simulink model "RobotAndBall"  (R2019b)
settings: Solver=VariableStepAuto  StartTime=0.0  StopTime=30  MaxStep=updateFrequency  RelTol=1e-3
values from neighbouring files (symbols this model uses):
  g = bTraj.GoalOnRight    [Launch_Game_TwoRobots.m]
  pOpponentSidePoint = [2.4;0;0.02]'    [Launch_Game_TwoRobots.m]
  Robot1 = RobotPlayer2(initialQ,TransMat1,DistToTable,'Left')    [Launch_Game_TwoRobots.m]
undefined symbols (not defined in the file or in its folder): Ball, Contact_Forces, currentTime, Environment, Net, Robots, Table, tHit, wayPoints, X, Y, Z
libraries: sm_lib x217, nesl_utility x89, Contact_Forces_Lib x8, robotmaniplib x8, Parts_Lib x6, Multibody_Parts_Lib x2, OpenManipulatorLib x1
(part 1 of 7)
settings Model: EnablePacing=on  Creator=Fadi  LastModifiedBy=Fadi
settings DebuggingCC: UnderSpecifiedDimensionMsg=warning
settings DiagnosticsConfigSet: SimMechanicsRigidlyBoundBlock=warning
settings ExplorerConfigSet: InternalSimMechanicsExplorerSettings="<ExplorerConfiguration><canonicalview>default</canonicalview><AnimationSetting><BasePlaybackSpeed>1.0</BasePlaybackSpeed><PlaybackSpeedFactor>1.0</PlaybackSpeedFactor></AnimationSetting><TilePanel><TileInfo><Tiles Columns=\"1\" Count=\"1\" Rows=\"1\"><Column Weight=\"1\"/><Row Weight=\"1\"/><Tile Height=\"1\" Width=\"1\" X=\"0\" Y=\"0\"/></Tiles></TileInfo><SceneInfo><SceneViewer><BGColor><R>0.800000011920928955</R><G>0.800000011920928955</G><B>0.800000011920928955</B></BGColor><Camera><DoPerspective>off</DoPerspective><Position><X>2.72315971629590692</X><Y>-1.50834696696562665</Y><Z>1.58535918834610445</Z></Position><Center><X>1.47795530502201444</X><Y>0.925758447867804257</Y><Z>-0.104613396829873029</Z></Center><Up><X>-0.0499239114255342065</X><Y>0.5522402253466272</Y><Z>0.832188882752636694</Z></Up><ViewLimDist>1</ViewLimDist><YLim>1.3965979297788147</YLim><XLim>2.09410606911342079</XLim></Camera></SceneViewer></SceneInfo></TilePanel><MechEditorPanel><Cameras><Camera><Id>Camera1</Id><Value><Name>Camera1</Name><NativeCamera><PositionTrackingFeature>Subsystem2.wall.R</PositionTrackingFeature><CenterTrackingFeature>Subsystem2.Sphere1.R</CenterTrackingFeature><UpVectorTrackingFeature>Subsystem2.Trans_Table_1.B</UpVectorTrackingFeature><CenterTrackingOrigin>on</CenterTrackingOrigin><UpVectorTrackingDirection>+Z</UpVectorTrackingDirection></NativeCamera></Value></Camera><Camera><Id>Camera2</Id><Value><Name>Camera2</Name><NativeCamera><PositionTrackingFeature>Subsystem2.Trans_Camera.F</PositionTrackingFeature><CenterTrackingFeature>Subsystem2.Sphere1.Sphere.R</CenterTrackingFeature><UpVectorTrackingFeature>Subsystem2.Subsystem1_Bottom</UpVectorTrackingFeature><CenterTrackingOrigin>on</CenterTrackingOrigin><UpVectorTrackingDirection>+Z</UpVectorTrackingDirection></NativeCamera></Value></Camera><Camera><Id>Camera3</Id><Value><Name>Camera3</Name><NativeCamera><PositionKeyframeSet><Keyframe><Time>0.092181068332948451</Time><Value><X>0.74195184319358032</X><Y>-2.1572930074306607</Y><Z>0.99365309767099308</Z></Value></Keyframe><Keyframe><Time>0.51650682316294461</Time><Value><X>1.9459936990787221</X><Y>-2.2708727878259349</Y><Z>1.6833699233296544</Z></Value></Keyframe><Keyframe><Time>0.91598798928248681</Time><Value><X>2.4643039101880788</X><Y>-0.44601289764194951</Y><Z>1.9211952797348746</Z></Value></Keyframe><Keyframe><Time>1.2186543181176928</Time><Value><X>3.2021539618459673</X><Y>0.10402512519052465</Y><Z>4.0341557316442129</Z></Value></Keyframe><Keyframe><Time>1.6120180307329675</Time><Value><X>1.47658917689103</X><Y>0.12690724272667403</Y><Z>3.9442623812733499</Z></Value></Keyframe></PositionKeyframeSet><CenterKeyframeSet><Keyframe><Time>0.092181068332948451</Time><Value><X>1.6664706896861596</X><Y>0.49901858600439208</Y><Z>0.12540780922655559</Z></Value></Keyframe><Keyframe><Time>0.51650682316294461</Time><Value><X>1.8354146075452522</X><Y>-0.67058112685808369</Y><Z>0.88017967418294973</Z></Value></Keyframe><Keyframe><Time>0.91598798928248681</Time><Value><X>1.6687021386666459</X><Y>0.49771837800342772</Y><Z>1.0348366085782759</Z></Value></Keyframe><Keyframe><Time>1.2186543181176928</Time><Value><X>1.8941663009838337</X><Y>1.0681539209099937</Y><Z>2.2215197753492841</Z></Value></Keyframe><Keyframe><Time>1.6120180307329675</Time><Value><X>1.47658917689103</X><Y>0.12690724272667403</Y><Z>-6.705520583238922e-10</Z></Value></Keyframe></CenterKeyframeSet><UpVectorKeyframeSet><Keyframe><Time>0.092181068332948451</Time><Value><X>-0.1061284820573538</X><Y>0.34211066924335759</Y><Z>0.93364716852034846</Z></Value></Keyframe><Keyframe><Time>0.51650682316294461</Time><Value><X>-0.21697539420554568</X><Y>0.42586969042681183</Y><Z>0.87838299453320468</Z></Value></Keyframe><Keyframe><Time>0.91598798928248681</Time><Value><X>-0.56097267127192785</X><Y>0.26399229177590544</Y><Z>0.78461310973558329</Z></Value></Keyframe><Keyframe><Time>1.2186543181176928</Time><Value><X>-0.77959242063363499</X><Y>0.10360787466061416</Y><Z>0.61765772560448062</Z></Value></Keyframe><Keyframe><Time>1.6120180307329675</Time><Value><X>-0.99999555996270595</X><Y>0.0029799420924429784</Y><Z>0</Z></Value></Keyframe></UpVectorKeyframeSet></NativeCamera></Value></Camera><Camera><Id>Camera4</Id><Value><Name>Camera4</Name><NativeCamera><PositionKeyframeSet><Keyframe><Time>0</Time><Value><X>1.634718226767613</X><Y>-3.0526201016665979</Y><Z>0.41798822769624983</Z></Value></Keyframe><Keyframe><Time>0.89165574668215009</Time><Value><X>1.7924264462253023</X><Y>-0.98308392755206742</Y><Z>0.55318583463515325</Z></Value></Keyframe><Keyframe><Time>1.6293434090182939</Time><Value><X>2.0909308885157523</X><Y>1.4458285342327477</Y><Z>2.7042868818040096</Z></Value></Keyframe><Keyframe><Time>2.0068297485509734</Time><Value><X>1.1851088199232986</X><Y>1.7025785749793547</Y><Z>1.9663502501044083</Z></Value></Keyframe><Keyframe><Time>2.3788243854617517</Time><Value><X>-0.73689322282398173</X><Y>1.0135139680640644</Y><Z>0.55257028629247507</Z></Value></Keyframe><Keyframe><Time>2.571358268924163</Time><Value><X>-0.88936881541680146</X><Y>0.54692833301781496</Y><Z>0.20169970252396985</Z></Value></Keyframe><Keyframe><Time>3.0017917048799663</Time><Value><X>-0.99378101342593106</X><Y>-0.88477660537923308</Y><Z>0.55083326620273587</Z></Value></Keyframe><Keyframe><Time>3.8286861711482381</Time><Value><X>1.7669783801752301</X><Y>-0.30065490623969737</Y><Z>0.48883711225906146</Z></Value></Keyframe><Keyframe><Time>4.2649999999999997</Time><Value><X>1.2845531289756482</X><Y>-1.1935311565853732</Y><Z>0.063513925983704644</Z></Value></Keyframe><Keyframe><Time>4.6495452085974227</Time><Value><X>1.2791670874978069</X><Y>-2.7978972452371327</Y><Z>0.18868794730739935</Z></Value></Keyframe><Keyframe><Time>4.9000000000000004</Time><Value><X>1.2995425546894361</X><Y>-3.357189246478486</Y><Z>0.070455084598260581</Z></Value></Keyframe><Keyframe><Time>5.6950000000000003</Time><Value><X>1.766827835394553</X><Y>-3.3830579189989827</Y><Z>0.16082327479556113</Z></Value></Keyframe></PositionKeyframeSet><CenterKeyframeSet><Keyframe><Time>0</Time><Value><X>1.6509000609385884</X><Y>-1.1240589910676677</Y><Z>0.40348620051772122</Z></Value></Keyframe><Keyframe><Time>0.89165574668215009</Time><Value><X>0.93615742103789701</X><Y>-0.20137995272314729</Y><Z>0.37829480091806594</Z></Value></Keyframe><Keyframe><Time>1.6293434090182939</Time><Value><X>2.0885972726581383</X><Y>0.24860742012283255</Y><Z>1.4063751490603302</Z></Value></Keyframe><Keyframe><Time>2.0068297485509734</Time><Value><X>1.5752094627651436</X><Y>0.22716215204440982</Y><Z>1.131274392808693</Z></Value></Keyframe><Keyframe><Time>2.3788243854617517</Time><Value><X>1.1917147713311742</X><Y>0.17399517479538895</Y><Z>0.78722645339598651</Z></Value></Keyframe><Keyframe><Time>2.571358268924163</Time><Value><X>1.1306706612540736</X><Y>0.090353502813585118</Y><Z>0.71978451413263045</Z></Value></Keyframe><Keyframe><Time>3.0017917048799663</Time><Value><X>1.1520318643377385</X><Y>-0.27369936990022159</Y><Z>0.77619141514906276</Z></Value></Keyframe><Keyframe><Time>3.8286861711482381</Time><Value><X>2.5989369494105272</X><Y>-0.016728058685721581</Y><Z>0.33602337998020815</Z></Value></Keyframe><Keyframe><Time>4.2649999999999997</Time><Value><X>1.8555061148079619</X><Y>-0.34348390445788701</Y><Z>0.58072340067093176</Z></Value></Keyframe><Keyframe><Time>4.6495452085974227</Time><Value><X>1.7851002621033936</X><Y>-1.039700189233455</Y><Z>0.6214864747415626</Z></Value></Keyframe><Keyframe><Time>4.9000000000000004</Time><Value><X>1.6628379347052082</X><Y>-1.3752973817880583</Y><Z>0.63505319457126874</Z></Value></Keyframe><Keyframe><Time>5.6950000000000003</Time><Value><X>1.8485025028194528</X><Y>-1.4197514343887292</Y><Z>0.65312080186801191</Z></Value></Keyframe></CenterKeyframeSet><UpVectorKeyframeSet><Keyframe><Time>0</Time><Value><X>0.0034928530200739921</X><Y>0.0074900458545164653</Y><Z>0.99996584901229379</Z></Value></Keyframe><Keyframe><Time>0.89165574668215009</Time><Value><X>-0.098674392407507278</X><Y>0.11310907107115013</Y><Z>0.98867067435240075</Z></Value></Keyframe><Keyframe><Time>1.6293434090182939</Time><Value><X>0.17649709441833861</X><Y>-0.72366247342212719</Y><Z>0.66720416682036177</Z></Value></Keyframe><Keyframe><Time>2.0068297485509734</Time><Value><X>0.2510236966651741</X><Y>-0.42568013653437631</Y><Z>0.86935811094889159</Z></Value></Keyframe><Keyframe><Time>2.3788243854617517</Time><Value><X>-0.050382070115773898</X><Y>0.15981873044644337</Y><Z>0.98585983811560973</Z></Value></Keyframe><Keyframe><Time>2.571358268924163</Time><Value><X>-0.20665101219239682</X><Y>0.17750955250842274</Y><Z>0.96217759167843731</Z></Value></Keyframe><Keyframe><Time>3.0017917048799663</Time><Value><X>-0.087913512557610485</X><Y>-0.058026130746536349</Y><Z>0.99443661560723362</Z></Value></Keyframe><Keyframe><Time>3.8286861711482381</Time><Value><X>0.17417095748939701</X><Y>0.019531148883155394</Y><Z>0.98452171727724258</Z></Value></Keyframe><Keyframe><Time>4.2649999999999997</Time><Value><X>-0.30033345042142284</X><Y>-0.34041414517873991</Y><Z>0.89102077883750297</Z></Value></Keyframe><Keyframe><Time>4.6495452085974227</Time><Value><X>-0.095137175335041818</X><Y>-0.21204376065752092</Y><Z>0.97261830202576671</Z></Value></Keyframe><Keyframe><Time>4.9000000000000004</Time><Value><X>-0.068234231430172015</X><Y>-0.26175041028570761</Y><Z>0.96272052662047136</Z></Value></Keyframe><Keyframe><Time>5.6950000000000003</Time><Value><X>-0.023020556104334601</X><Y>-0.24225394172083331</Y><Z>0.96993973097165509</Z></Value></Keyframe></UpVectorKeyframeSet></NativeCamera></Value></Camera></Cameras><GfxPanelCameraMap/><VideoCreator><PlaybackSpeedRatio>0.25</PlaybackSpeedRatio><FrameRate>60</FrameRate><VideoFormat>MPEG-4</VideoFormat><FrameSize>auto</FrameSize></VideoCreator></MechEditorPanel></ExplorerConfiguration>"

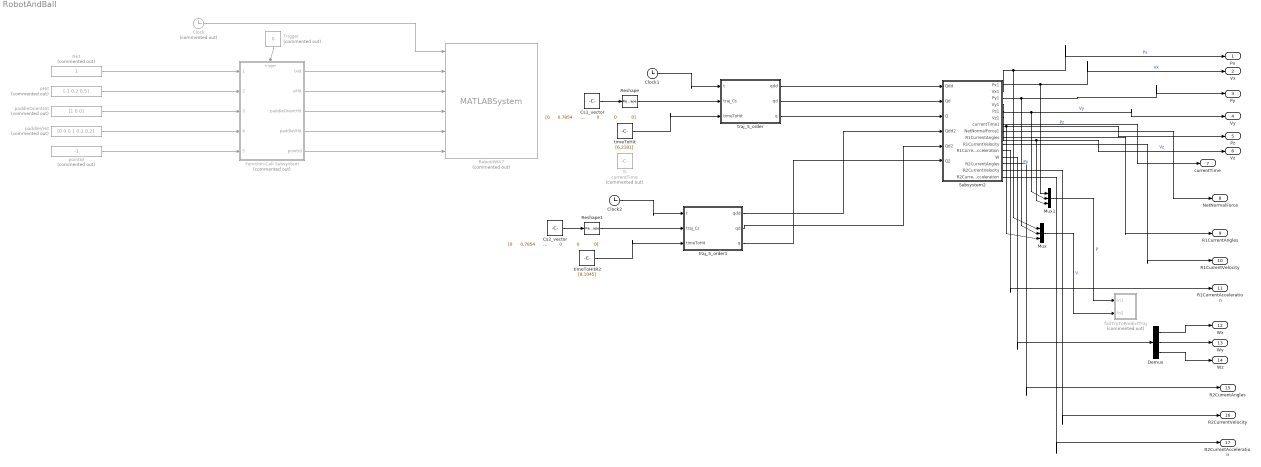
== system RobotAndBall ==
  Clock : Clock  Commented=on
  Clock1 : Clock
  Clock2 : Clock
  Cs1_vector : Constant  Value="[0      0.7854           0     -0.7854           0      1.5708           0           0           0           0           0           0           0           0           0           0           0           0           0           0           0           0           0           0           0           0           0           0           0           0           0           0           0           0           0           0           0           0           0           0           0           0]"  SampleTime=0.005
  Cs2_vector : Constant  Value="[0      0.7854           0     -0.7854           0      1.5708           0           0           0           0           0           0           0           0           0           0           0           0           0           0           0           0           0           0           0           0           0           0           0           0           0           0           0           0           0           0           0           0           0           0           0           0]"  SampleTime=0.005
  Demux : Demux  Outputs=3
  Function-Call Subsystem : Subsystem  Commented=on  TreatAsAtomicUnit=on
  Mux : Mux  Inputs=3
  Mux1 : Mux  Inputs=3
  Reshape : Reshape  OutputDimensionality=Customize  OutputDimensions=[7,6]
  Reshape1 : Reshape  OutputDimensionality=Customize  OutputDimensions=[7,6]
  RobotIIWA7 : MATLABSystem  Commented=on  System=RobotIIWA7  initialQ=[ 0, pi / 4, 0, -pi / 4, 0, pi / 4, 0 ]'  SimulateUsing=Interpreted execution
      mask Type: RobotIIWA7
      mask Display:
      | disp('RobotIIWA7');
      | port_label('input',1,'t');
      | port_label('input',2,'tHit');
      | port_label('input',3,'pHit');
      | port_label('input',4,'paddleOrientHit');
      | port_label('input',5,'paddleVHit');
      | port_label('input',6,'id');
      | port_label('output',1,'q');
      | port_label('output',2,'qd');
      | port_label('output',3,'qdd');
  Subsystem2 : Subsystem
  Ti : Constant  Commented=on  Value=currentTime
  Trigger : Constant  Commented=on  Value=0
  failTryToPredictTraj : Subsystem  Commented=on
  pHit : Constant  Commented=on  Value=[-1 0.2 0.5]
  paddleOrientHit : Constant  Commented=on  Value=[1 0 0]
  paddleVHit : Constant  Commented=on  Value=[0 0 0 1 0.1 0.2]
  pointId : Constant  Commented=on  Value=-1  OutDataTypeStr=Inherit: Inherit via back propagation
  tHit : Constant  Commented=on
  timeToHit : Constant  Value=[6.2181]
  timeToHitR2 : Constant  Value=[8.1045]
  traj_5_order : MATLAB Function  TreatAsAtomicUnit=on
  traj_5_order1 : MATLAB Function  TreatAsAtomicUnit=on
  Px : Outport
  Vx : Outport  Port=2
  Py : Outport  Port=3
  Vy : Outport  Port=4
  Pz : Outport  Port=5
  Vz : Outport  Port=6
  currentTime : Outport  Port=7
  NetNormalForce : Outport  Port=8
  R1CurrentAngles : Outport  Port=9
  R1CurrentVelocity : Outport  Port=10
  R1CurrentAcceleration : Outport  Port=11
  Wx : Outport  Port=12
  Wy : Outport  Port=13
  Wz : Outport  Port=14
  R2CurrentAngles : Outport  Port=15
  R2CurrentVelocity : Outport  Port=16
  R2CurrentAcceleration : Outport  Port=17
  wires:
  Subsystem2/4(Vy1) -> Vy/1, Mux1/2  "Vy"
  Subsystem2/5(Pz1) -> Pz/1, Mux/3  "Pz"
  Subsystem2/3(Py1) -> Py/1, Mux/2  "Py"
  Subsystem2/1(Px1) -> Mux/1, Px/1  "Px"
  Subsystem2/6(Vz1) -> Vz/1, Mux1/3  "Vz"
  Subsystem2/2(Vx1) -> Mux1/1, Vx/1  "Vx"
  Subsystem2/7(currentTime1) -> currentTime/1
  Subsystem2/8(NetNormalForce1) -> NetNormalForce/1
  Mux1/1 -> failTryToPredictTraj/1(In1)  "P"
  Mux/1 -> failTryToPredictTraj/2(In2)  "V"
  Trigger/1 -> Function-Call Subsystem/Trigger
  Clock/1 -> RobotIIWA7/1
  tHit/1 -> Function-Call Subsystem/1(1)
  pHit/1 -> Function-Call Subsystem/2(2)
  paddleOrientHit/1 -> Function-Call Subsystem/3(3)
  paddleVHit/1 -> Function-Call Subsystem/4(4)
  pointId/1 -> Function-Call Subsystem/5(5)
  Function-Call Subsystem/1(tHit) -> RobotIIWA7/2
  Function-Call Subsystem/2(pHit) -> RobotIIWA7/3
  Function-Call Subsystem/3(paddleOrientHit) -> RobotIIWA7/4
  Function-Call Subsystem/4(paddleVHit) -> RobotIIWA7/5
  Function-Call Subsystem/5(pointId) -> RobotIIWA7/6
  Subsystem2/9(R1CurrentAngles) -> R1CurrentAngles/1
  Subsystem2/10(R1CurrentVelocity) -> R1CurrentVelocity/1
  Subsystem2/11(R1CurrentAcceleration) -> R1CurrentAcceleration/1
  Clock1/1 -> traj_5_order/1(t)
  Cs1_vector/1 -> Reshape/1
  Reshape/1 -> traj_5_order/2(traj_Cs)
  traj_5_order/1(qdd) -> Subsystem2/1(Qdd)
  traj_5_order/2(qd) -> Subsystem2/2(Qd)
  traj_5_order/3(q) -> Subsystem2/3(Q)
  timeToHit/1 -> traj_5_order/3(timeToHit)
  Demux/1 -> Wx/1
  Demux/2 -> Wy/1
  Demux/3 -> Wz/1
  Subsystem2/12(W) -> Demux/1
  traj_5_order1/3(q) -> Subsystem2/6(Q2)
  timeToHitR2/1 -> traj_5_order1/3(timeToHit)
  traj_5_order1/2(qd) -> Subsystem2/5(Qd2)
  Cs2_vector/1 -> Reshape1/1
  Reshape1/1 -> traj_5_order1/2(traj_Cs)
  traj_5_order1/1(qdd) -> Subsystem2/4(Qdd2)
  Clock2/1 -> traj_5_order1/1(t)
  Subsystem2/13(R2CurrentAngles) -> R2CurrentAngles/1
  Subsystem2/14(R2CurrentVelocity) -> R2CurrentVelocity/1
  Subsystem2/15(R2CurrentAcceleration) -> R2CurrentAcceleration/1

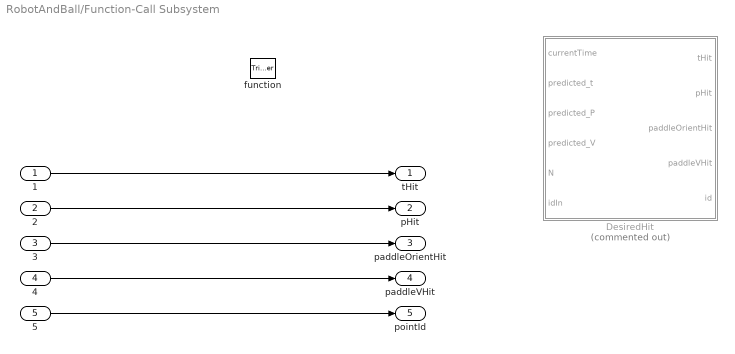
== system RobotAndBall/Function-Call Subsystem ==
  1 : Inport
  2 : Inport  Port=2
  3 : Inport  Port=3
  4 : Inport  Port=4
  5 : Inport  Port=5
  function : TriggerPort  TriggerType=either  VariantControl=Variant
  DesiredHit : MATLAB Function  Commented=on  TreatAsAtomicUnit=on
  tHit : Outport  PortDimensions=1
  pHit : Outport  Port=2  PortDimensions=3
  paddleOrientHit : Outport  Port=3  PortDimensions=3
  paddleVHit : Outport  Port=4  PortDimensions=6
  pointId : Outport  Port=5
  wires:
  1/1 -> tHit/1
  4/1 -> paddleVHit/1
  3/1 -> paddleOrientHit/1
  2/1 -> pHit/1
  5/1 -> pointId/1
